simulink model "swerve_steering_unit_sim"  (R2023b)
settings: Solver=VariableStepDiscrete  StartTime=0.0  StopTime=4  MaxStep=.02  RelTol=1e-3
undefined symbols (not defined in the file): AT_Yaw_Control_Gain, DiscIntNeverNeededParam, Steering_Abs_Deadband_Range, Steering_Cmd_Timeout, Steering_Mod_Str_Rel_in, Steering_Mod_Str_Rel_out, Steering_Relative_Gain, Steering_Twist_Gain
libraries: simulink x11, hdlsllib x5
settings Model: Creator=ander  LastModifiedBy=ander

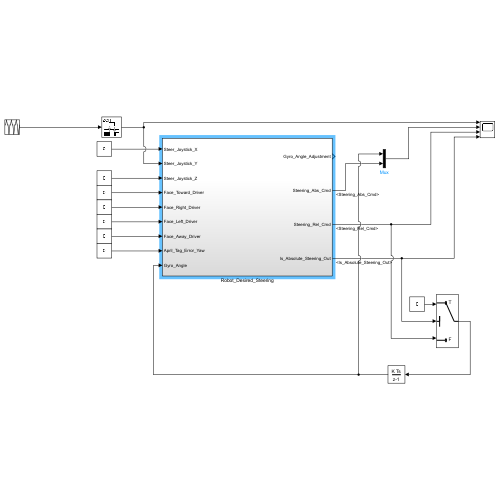
[thumbnail: Simulink's stored preview of the top-level diagram]
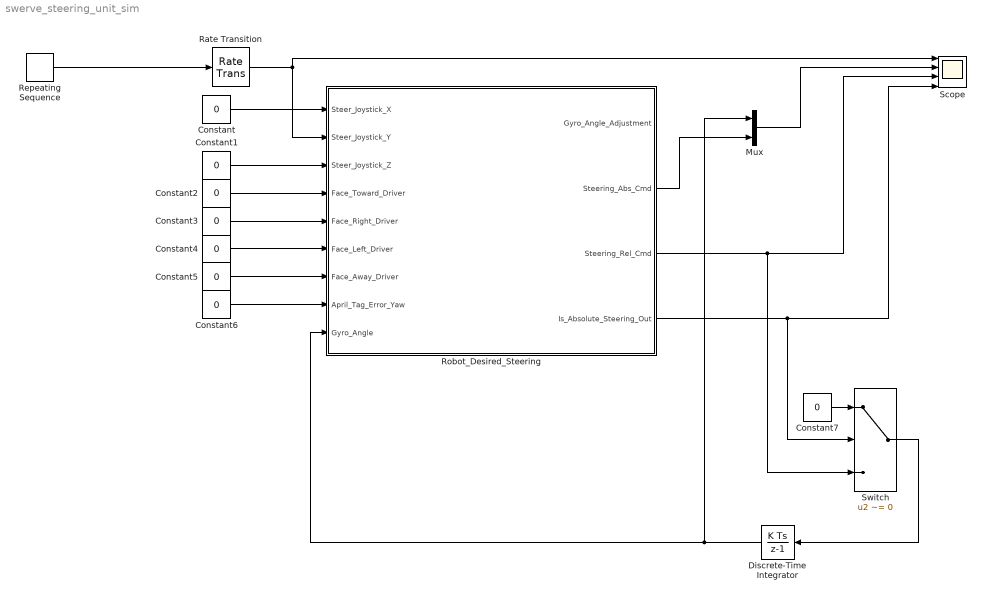
== system swerve_steering_unit_sim ==
  Constant{,1..7} (8 alike) : Constant  Value=0
  Discrete-Time Integrator : DiscreteIntegrator  gainval=0.2  SampleTime=-1  ICPrevOutput=DiscIntNeverNeededParam  ICPrevScaledInput=DiscIntNeverNeededParam
  Mux : Mux  Inputs=2
  Rate Transition : RateTransition  OutPortSampleTime=0.02
  Repeating Sequence : simulink/Sources/Repeating Sequence  rep_seq_t=[0 0.1 1 1.9 2.1 3 3.9 4.1]  rep_seq_y=[0 0 1 0 0 -2 0 0]
  Robot_Desired_Steering : Subsystem
  Scope : Scope  NumInputPorts=4
  Switch : Switch  Criteria=u2 ~= 0  SaturateOnIntegerOverflow=off  InputSameDT=off
  wires:
  Constant1/1 -> Robot_Desired_Steering/3(Steer_Joystick_Z)
  Constant2/1 -> Robot_Desired_Steering/4(Face_Toward_Driver)
  Constant3/1 -> Robot_Desired_Steering/5(Face_Right_Driver)
  Constant4/1 -> Robot_Desired_Steering/6(Face_Left_Driver)
  Constant5/1 -> Robot_Desired_Steering/7(Face_Away_Driver)
  Constant6/1 -> Robot_Desired_Steering/8(April_Tag_Error_Yaw)
  Rate Transition/1 -> Robot_Desired_Steering/2(Steer_Joystick_Y), Scope/1
  Robot_Desired_Steering/3(Steering_Rel_Cmd) -> Switch/3, Scope/3
  Robot_Desired_Steering/4(Is_Absolute_Steering_Out) -> Switch/2, Scope/4
  Repeating Sequence/1 -> Rate Transition/1
  Constant/1 -> Robot_Desired_Steering/1(Steer_Joystick_X)
  Mux/1 -> Scope/2
  Robot_Desired_Steering/2(Steering_Abs_Cmd) -> Mux/2
  Constant7/1 -> Switch/1
  Switch/1 -> Discrete-Time Integrator/1
  Discrete-Time Integrator/1 -> Mux/1, Robot_Desired_Steering/9(Gyro_Angle)

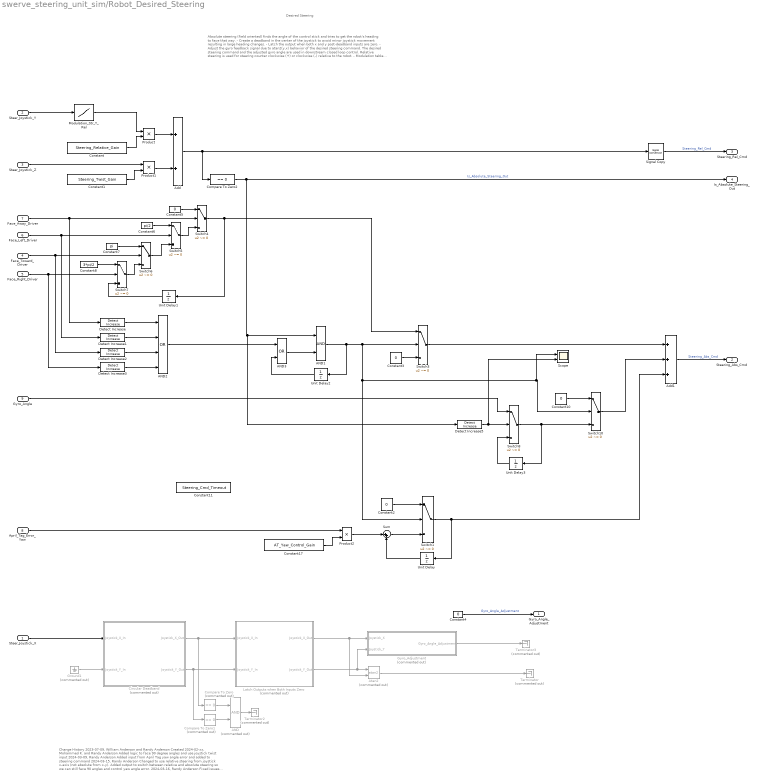
== system swerve_steering_unit_sim/Robot_Desired_Steering ==
  note: Change History
      | 2023-07-09, William Anderson and Randy Anderson
      | Created
      | 2024-02-xx, Mohammed K. and Randy Anderson
      | Added logic to face 90 degree angles and use joystick twist input
      | 2024-03-09, Randy Anderson
      | Added input from April Tag yaw angle error and added to steering command
      | 2024-03-15, Randy Anderson
      | Changed to use relative steering from joystick x-axis (not absolute from x-y).
      | Added output to switch between relative and absolute steering so we can still
      | face 90 angles and control yaw angle error.
      | 2024-03-16, Randy Anderson
      | Fixed issues with using yaw error and snapping to 90 degree angles when
      | coupled with relative steering.
      | 2024-03-18, Randy Anderosn
      | Added gyro angle input to make corrections to robot heading while driving
      | without driver steering input.
  note: Desired Steering
  note: Absolute steering (field oriented) finds the angle of the control stick and tries to get the robot's heading to face that way.
      | - Create a deadband in the center of the joystick to avoid minor joystick movement resulting in large heading changes.
      | - Latch the output when both x and y post-deadband inputs are zero.
      | - Adjust the gyro feedback signal due to atan2(y,x) behavior of the desired steering command. The desired steering command and the adjusted gyro angle are used in downstream closed loop control.
      |
      | Relative steering is used for steering counter clockwise (+) or clockwise (-) relative to the robot.
      | - Modulation table for joystick input. Only one axis of the steering joystck is used.
      | - The gain block adjusts how fast the robot will rotate.
      |
      | NEED TO UPDATE
  Steer_Joystick_X : Inport
  Steer_Joystick_Y : Inport  Port=2
  Steer_Joystick_Z : Inport  Port=3
  Face_Toward_Driver : Inport  Port=4
  Face_Right_Driver : Inport  Port=5
  Face_Left_Driver : Inport  Port=6
  Face_Away_Driver : Inport  Port=7
  April_Tag_Error_Yaw : Inport  Port=8
  Gyro_Angle : Inport  Port=9
  AND : Logic  Commented=on  AllPortsSameDT=off  OutDataTypeStr=boolean
  AND1 : Logic  AllPortsSameDT=off  OutDataTypeStr=boolean
  AND2 : Logic  Operator=OR  Inputs=4  AllPortsSameDT=off  OutDataTypeStr=boolean
  AND3 : Logic  Operator=OR  AllPortsSameDT=off  OutDataTypeStr=boolean
  Add : Sum
  Add1 : Sum  Inputs=3
  Atan2 : Trigonometry  Commented=on  Operator=atan2
  Circular Deadband : Subsystem  Commented=on
  Compare To Zero : simulink/Logic and Bit Operations/Compare To Zero  Commented=on  relop===  OutDataTypeStr=boolean
  Compare To Zero1 : simulink/Logic and Bit Operations/Compare To Zero  Commented=on  relop===  OutDataTypeStr=boolean
  Compare To Zero2 : simulink/Logic and Bit Operations/Compare To Zero  relop===  OutDataTypeStr=boolean
  Constant : Constant  Value=Steering_Relative_Gain
  Constant1 : Constant  Value=Steering_Twist_Gain
  Constant{2..5,10} (5 alike) : Constant  Value=0
  Constant11 : Constant  Value=Steering_Cmd_Timeout
  Constant17 : Constant  Value=AT_Yaw_Control_Gain
  Constant6 : Constant  Value=pi/2
  Constant7 : Constant  Value=pi
  Constant8 : Constant  Value=3*pi/2
  Detect Increase{,1..3,5} (5 alike) : simulink/Logic and Bit Operations/Detect Increase  vinit=0.0  OutDataTypeStr=boolean
  Ground1 : Ground  Commented=on
  Gyro_Adjustment : Subsystem  Commented=on
  Latch Outputs when Both Inputs Zero : Subsystem  Commented=on
  Modulation_Str_Y_Rel : Lookup_n-D  NumberOfTableDimensions=1  BreakpointsForDimension1=Steering_Mod_Str_Rel_in  Table=Steering_Mod_Str_Rel_out  ExtrapMethod=Clip  InternalRulePriority=Speed  RndMeth=Simplest
  Product : Product
  Product1 : Product
  Product2 : Product
  Scope : Scope  NumInputPorts=2
  Signal Copy : SignalConversion  OverrideOpt=off
  Sum : Sum  Inputs=|++
  Switch{1,3..8,10} (8 alike) : Switch  Criteria=u2 ~= 0  SaturateOnIntegerOverflow=off  InputSameDT=off
  Terminator : Terminator  Commented=on
  Terminator2 : Terminator  Commented=on
  Terminator3 : Terminator  Commented=on
  Unit Delay{,1..3} (4 alike) : UnitDelay  SampleTime=-1  HasFrameUpgradeWarning=on
  Gyro_Angle_Adjustment : Outport
  Steering_Abs_Cmd : Outport  Port=2
  Steering_Rel_Cmd : Outport  Port=3
  Is_Absolute_Steering_Out : Outport  Port=4
  wires:
  Product2/1 -> Sum/1
  Constant2/1 -> Switch1/1
  Unit Delay/1 -> Sum/2
  Sum/1 -> Switch1/3
  Switch10/1 -> Add1/2
  Steer_Joystick_Y/1 -> Modulation_Str_Y_Rel/1
  Detect Increase5/1 -> Scope/2, Switch8/2
  Unit Delay3/1 -> Switch8/3
  Switch8/1 -> Unit Delay3/1, Switch10/3
  Gyro_Angle/1 -> Switch8/1
  Switch3/1 -> Add1/1
  Constant3/1 -> Switch3/3
  Add1/1 -> Steering_Abs_Cmd/1  "Steering_Abs_Cmd"
  Product1/1 -> Add/2
  Product/1 -> Add/1
  Steer_Joystick_X/1 -> Circular Deadband/1(Joystick_X_In)
  Ground1/1 -> Circular Deadband/2(Joystick_Y_In)
  Gyro_Adjustment/1(Gyro_Angle_Adjustment) -> Terminator3/1
  Face_Right_Driver/1 -> Detect Increase3/1, Switch7/2
  Face_Toward_Driver/1 -> Detect Increase2/1, Switch6/2
  Face_Left_Driver/1 -> Detect Increase1/1, Switch5/2
  Face_Away_Driver/1 -> Detect Increase/1, Switch4/2
  Switch7/1 -> Switch6/3
  Switch5/1 -> Switch4/3
  Constant8/1 -> Switch7/1
  Constant6/1 -> Switch5/1
  Switch6/1 -> Switch5/3
  Constant7/1 -> Switch6/1
  Constant5/1 -> Switch4/1
  Constant1/1 -> Product1/2
  Switch1/1 -> Add1/3, Unit Delay/1
  Compare To Zero1/1 -> AND/2
  Compare To Zero/1 -> AND/1
  Steer_Joystick_Z/1 -> Product1/1
  Modulation_Str_Y_Rel/1 -> Product/1
  Add/1 -> Compare To Zero2/1, Signal Copy/1
  Constant/1 -> Product/2
  Constant4/1 -> Gyro_Angle_Adjustment/1  "Gyro_Angle_Adjustment"
  Latch Outputs when Both Inputs Zero/2(Joystick_Y_Out) -> Gyro_Adjustment/2(Joystick_Y), Atan2/1
  Circular Deadband/2(Joystick_Y_Out) -> Compare To Zero1/1, Latch Outputs when Both Inputs Zero/2(Joystick_Y_In)
  Circular Deadband/1(Joystick_X_Out) -> Latch Outputs when Both Inputs Zero/1(Joystick_X_In), Compare To Zero/1
  Latch Outputs when Both Inputs Zero/1(Joystick_X_Out) -> Atan2/2, Gyro_Adjustment/1(Joystick_X)
  Switch4/1 -> Unit Delay1/1, Switch3/1
  Unit Delay1/1 -> Switch7/3
  AND1/1 -> Scope/1, Switch10/2, Switch1/2, Switch3/2, Unit Delay2/1
  Detect Increase/1 -> AND2/1
  Detect Increase1/1 -> AND2/2
  Detect Increase2/1 -> AND2/3
  Detect Increase3/1 -> AND2/4
  AND2/1 -> AND3/1
  AND3/1 -> AND1/2
  Unit Delay2/1 -> AND3/2
  Constant17/1 -> Product2/2
  April_Tag_Error_Yaw/1 -> Product2/1
  Atan2/1 -> Terminator/1
  Compare To Zero2/1 -> Detect Increase5/1, AND1/1, Is_Absolute_Steering_Out/1  "Is_Absolute_Steering_Out"
  AND/1 -> Terminator2/1
  Signal Copy/1 -> Steering_Rel_Cmd/1  "Steering_Rel_Cmd"
  Constant10/1 -> Switch10/1

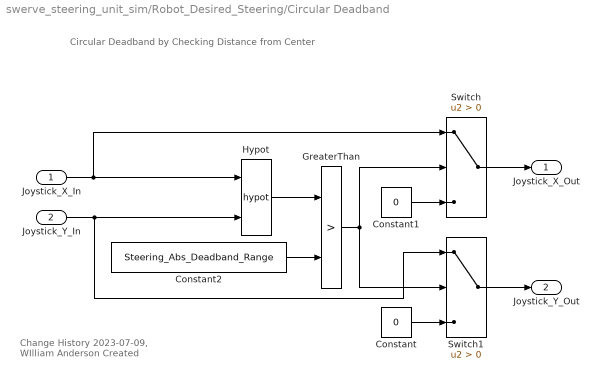
== system swerve_steering_unit_sim/Robot_Desired_Steering/Circular Deadband ==
  note: Change History
      | 2023-07-09, WIlliam Anderson
      | Created
  note: Circular Deadband by Checking Distance from Center
  Joystick_X_In : Inport
  Joystick_Y_In : Inport  Port=2
  Constant : Constant  Value=0
  Constant1 : Constant  Value=0
  Constant2 : Constant  Value=Steering_Abs_Deadband_Range
  GreaterThan : RelationalOperator  Operator=>  OutDataTypeStr=boolean  RndMeth=Simplest  InputSameDT=off
  Hypot : Math  Operator=hypot
  Switch : Switch  Criteria=u2 > Threshold  SaturateOnIntegerOverflow=off  InputSameDT=off
  Switch1 : Switch  Criteria=u2 > Threshold  SaturateOnIntegerOverflow=off  InputSameDT=off
  Joystick_X_Out : Outport
  Joystick_Y_Out : Outport  Port=2
  wires:
  Switch1/1 -> Joystick_Y_Out/1
  Switch/1 -> Joystick_X_Out/1
  Constant/1 -> Switch1/3
  Constant1/1 -> Switch/3
  Joystick_X_In/1 -> Hypot/1, Switch/1
  Joystick_Y_In/1 -> Switch1/1, Hypot/2
  Hypot/1 -> GreaterThan/1
  Constant2/1 -> GreaterThan/2
  GreaterThan/1 -> Switch/2, Switch1/2

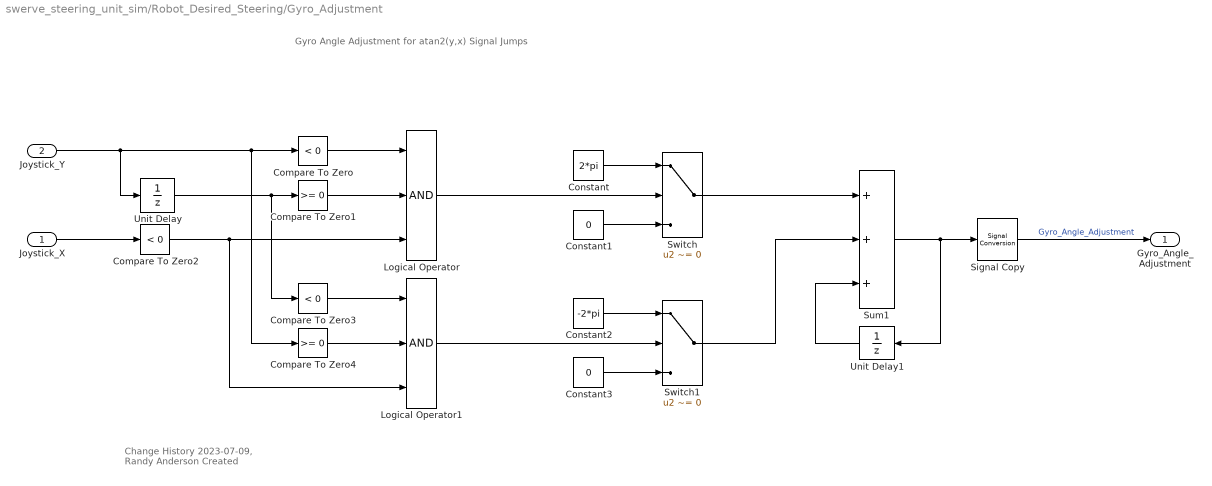
== system swerve_steering_unit_sim/Robot_Desired_Steering/Gyro_Adjustment ==
  note: Change History
      | 2023-07-09, Randy Anderson
      | Created
  note: Gyro Angle Adjustment for atan2(y,x) Signal Jumps
  Joystick_X : Inport
  Joystick_Y : Inport  Port=2
  Compare To Zero : hdlsllib/Logic and Bit Operations/Compare To Zero  relop=<  OutDataTypeStr=boolean
  Compare To Zero1 : hdlsllib/Logic and Bit Operations/Compare To Zero  relop=>=  OutDataTypeStr=boolean
  Compare To Zero2 : hdlsllib/Logic and Bit Operations/Compare To Zero  relop=<  OutDataTypeStr=boolean
  Compare To Zero3 : hdlsllib/Logic and Bit Operations/Compare To Zero  relop=<  OutDataTypeStr=boolean
  Compare To Zero4 : hdlsllib/Logic and Bit Operations/Compare To Zero  relop=>=  OutDataTypeStr=boolean
  Constant : Constant  Value=2*pi
  Constant1 : Constant  Value=0
  Constant2 : Constant  Value=-2*pi
  Constant3 : Constant  Value=0
  Logical Operator : Logic  Inputs=3  AllPortsSameDT=off  OutDataTypeStr=boolean
  Logical Operator1 : Logic  Inputs=3  AllPortsSameDT=off  OutDataTypeStr=boolean
  Signal Copy : SignalConversion  OverrideOpt=off
  Sum1 : Sum  Inputs=3
  Switch : Switch  Criteria=u2 ~= 0  SaturateOnIntegerOverflow=off  InputSameDT=off
  Switch1 : Switch  Criteria=u2 ~= 0  SaturateOnIntegerOverflow=off  InputSameDT=off
  Unit Delay : UnitDelay  SampleTime=-1  HasFrameUpgradeWarning=on
  Unit Delay1 : UnitDelay  SampleTime=-1  HasFrameUpgradeWarning=on
  Gyro_Angle_Adjustment : Outport
  wires:
  Signal Copy/1 -> Gyro_Angle_Adjustment/1  "Gyro_Angle_Adjustment"
  Switch1/1 -> Sum1/2
  Constant2/1 -> Switch1/1
  Constant3/1 -> Switch1/3
  Logical Operator1/1 -> Switch1/2
  Compare To Zero4/1 -> Logical Operator1/2
  Compare To Zero3/1 -> Logical Operator1/1
  Compare To Zero2/1 -> Logical Operator/3, Logical Operator1/3
  Joystick_X/1 -> Compare To Zero2/1
  Unit Delay1/1 -> Sum1/3
  Switch/1 -> Sum1/1
  Sum1/1 -> Signal Copy/1, Unit Delay1/1
  Logical Operator/1 -> Switch/2
  Constant1/1 -> Switch/3
  Constant/1 -> Switch/1
  Compare To Zero1/1 -> Logical Operator/2
  Compare To Zero/1 -> Logical Operator/1
  Unit Delay/1 -> Compare To Zero1/1, Compare To Zero3/1
  Joystick_Y/1 -> Unit Delay/1, Compare To Zero/1, Compare To Zero4/1

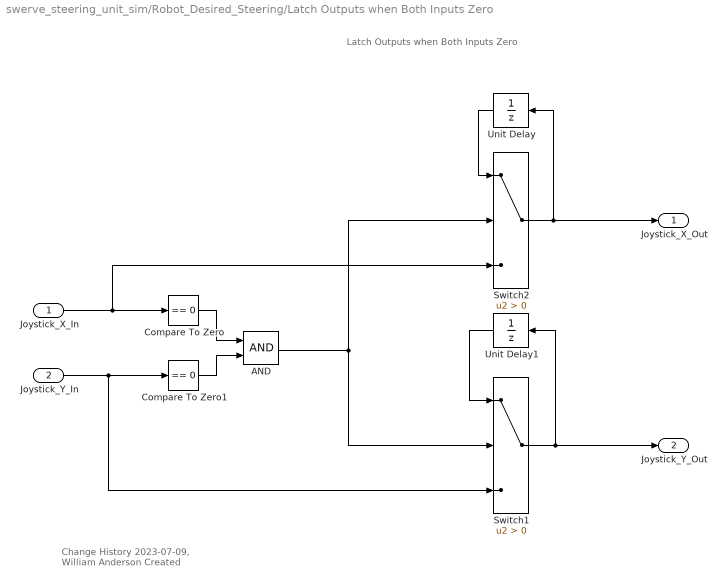
== system swerve_steering_unit_sim/Robot_Desired_Steering/Latch Outputs when Both Inputs Zero ==
  note: Change History
      | 2023-07-09, William Anderson
      | Created
  note: Latch Outputs when Both Inputs Zero
  Joystick_X_In : Inport
  Joystick_Y_In : Inport  Port=2
  AND : Logic  AllPortsSameDT=off  OutDataTypeStr=boolean
  Compare To Zero : simulink/Logic and Bit Operations/Compare To Zero  relop===  OutDataTypeStr=boolean
  Compare To Zero1 : simulink/Logic and Bit Operations/Compare To Zero  relop===  OutDataTypeStr=boolean
  Switch1 : Switch  Criteria=u2 > Threshold  SaturateOnIntegerOverflow=off  InputSameDT=off
  Switch2 : Switch  Criteria=u2 > Threshold  SaturateOnIntegerOverflow=off  InputSameDT=off
  Unit Delay : UnitDelay  SampleTime=-1  HasFrameUpgradeWarning=on
  Unit Delay1 : UnitDelay  SampleTime=-1  HasFrameUpgradeWarning=on
  Joystick_X_Out : Outport
  Joystick_Y_Out : Outport  Port=2
  wires:
  Switch1/1 -> Joystick_Y_Out/1, Unit Delay1/1
  Switch2/1 -> Joystick_X_Out/1, Unit Delay/1
  Joystick_X_In/1 -> Switch2/3, Compare To Zero/1
  Joystick_Y_In/1 -> Switch1/3, Compare To Zero1/1
  Compare To Zero1/1 -> AND/2
  Compare To Zero/1 -> AND/1
  AND/1 -> Switch1/2, Switch2/2
  Unit Delay/1 -> Switch2/1
  Unit Delay1/1 -> Switch1/1
